simulink subsystem "CompAbs"  (R2023b)
settings: Solver=VariableStepAuto  StartTime=0.0  StopTime=10.0  RelTol=1e-3
settings Model: Creator=Koche  LastModifiedBy=Koche

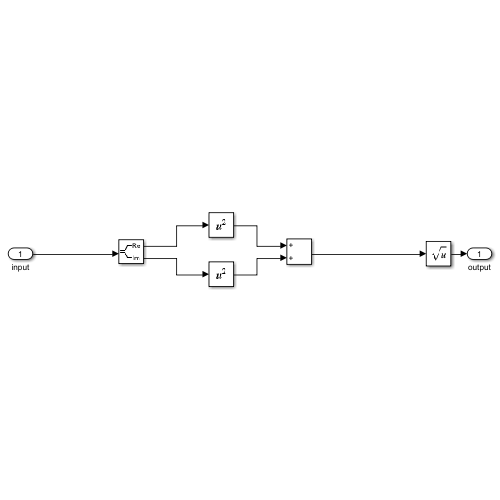
[thumbnail: Simulink's stored preview of the top-level diagram]
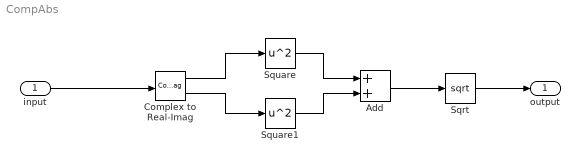
== system CompAbs ==
  input : Inport
  Add : Sum
  Complex to Real-Imag : ComplexToRealImag
  Sqrt : Sqrt
  Square : Math  Operator=square  SignedPower=on  RndMeth=Zero
  Square1 : Math  Operator=square  SignedPower=on  RndMeth=Zero
  output : Outport
  wires:
  input/1 -> Complex to Real-Imag/1
  Sqrt/1 -> output/1
  Square/1 -> Add/1
  Complex to Real-Imag/1 -> Square/1
  Square1/1 -> Add/2
  Add/1 -> Sqrt/1
  Complex to Real-Imag/2 -> Square1/1
